simulink model "Old Observer"  (R2022a)
settings: Solver=VariableStepAuto  StartTime=0  StopTime=1000  RelTol=1e-3
undefined symbols (not defined in the file): A_HD, A_platform, B_HD, B_platform, C_HD, C_platform, E_platform, L_platform, P_platform, Q_platform
settings Model: Creator=ianam  LastModifiedBy=ianam
settings DebuggingCC: UnderSpecifiedDataTypeMsg=error  UnderSpecifiedDimensionMsg=error

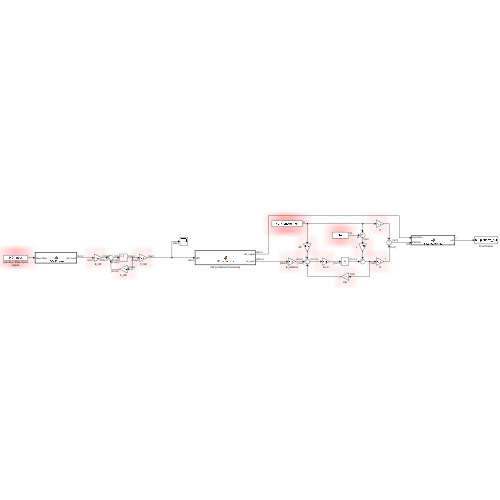
[thumbnail: Simulink's stored preview of the top-level diagram]
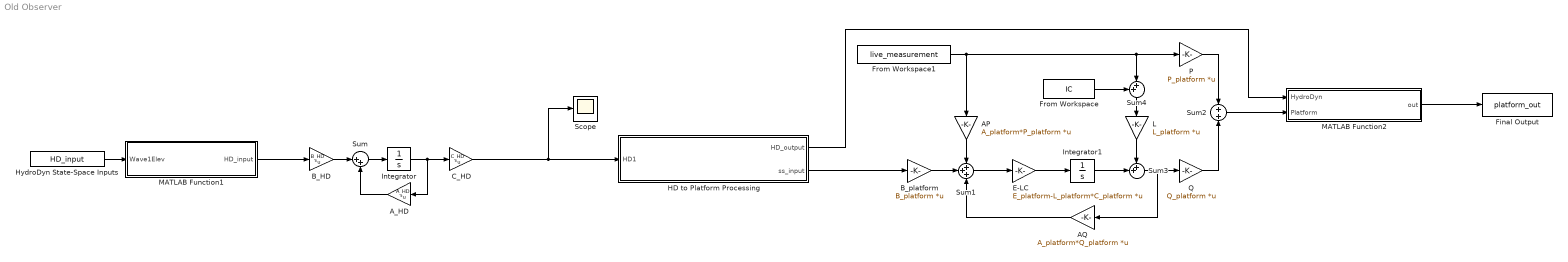
== system Old Observer ==
  AP : Gain  Gain=A_platform*P_platform  Multiplication=Matrix(K*u)
  AQ : Gain  Gain=A_platform*Q_platform  Multiplication=Matrix(K*u)
  A_HD : Gain  Gain=A_HD  Multiplication=Matrix(K*u)
  B_HD : Gain  Gain=B_HD  Multiplication=Matrix(K*u)
  B_platform : Gain  Gain=B_platform  Multiplication=Matrix(K*u)
  C_HD : Gain  Gain=C_HD  Multiplication=Matrix(K*u)
  E-LC : Gain  Gain=E_platform-L_platform*C_platform  Multiplication=Matrix(K*u)
  Final Output : ToWorkspace  VariableName=platform_out  SaveFormat=Timeseries  SampleTime=-1
  From Workspace : FromWorkspace  VariableName=IC
  From Workspace1 : FromWorkspace  VariableName=live_measurement
  HD to Platform Processing : MATLAB Function  TreatAsAtomicUnit=on
  HydroDyn State-Space Inputs : FromWorkspace  VariableName=HD_input
  Integrator : Integrator
  Integrator1 : Integrator
  L : Gain  Gain=L_platform  Multiplication=Matrix(K*u)
  MATLAB Function1 : MATLAB Function  TreatAsAtomicUnit=on
  MATLAB Function2 : MATLAB Function  TreatAsAtomicUnit=on
  P : Gain  Gain=P_platform  Multiplication=Matrix(K*u)
  Q : Gain  Gain=Q_platform  Multiplication=Matrix(K*u)
  Scope : Scope
  Sum : Sum  Inputs=|++
  Sum1 : Sum  Inputs=+++
  Sum2 : Sum  Inputs=+|+
  Sum3 : Sum  Inputs=++|
  Sum4 : Sum  Inputs=++|
  wires:
  Sum/1 -> Integrator/1
  Integrator/1 -> C_HD/1, A_HD/1
  A_HD/1 -> Sum/2
  B_HD/1 -> Sum/1
  MATLAB Function1/1(HD_input) -> B_HD/1
  HD to Platform Processing/2(ss_input) -> B_platform/1
  HydroDyn State-Space Inputs/1 -> MATLAB Function1/1(Wave1Elev)
  C_HD/1 -> Scope/1, HD to Platform Processing/1(HD1)
  AQ/1 -> Sum1/3
  B_platform/1 -> Sum1/2
  Sum1/1 -> E-LC/1
  E-LC/1 -> Integrator1/1
  AP/1 -> Sum1/1
  From Workspace1/1 -> P/1, Sum4/2, AP/1
  From Workspace/1 -> Sum4/1
  Integrator1/1 -> Sum3/2
  Sum4/1 -> L/1
  L/1 -> Sum3/1
  Sum3/1 -> AQ/1, Q/1
  P/1 -> Sum2/1
  Q/1 -> Sum2/2
  HD to Platform Processing/1(HD_output) -> MATLAB Function2/1(HydroDyn)
  Sum2/1 -> MATLAB Function2/2(Platform)
  MATLAB Function2/1(out) -> Final Output/1

== matlab function Old Observer/MATLAB Function1 ==
  data: Wave1Elev input; HD_input output
function HD_input = HDOutProcess(Wave1Elev)

% Create input vector
HD_input = zeros(37,1);

% Assign HD outputs to input vector
HD_input(37) = Wave1Elev;

end

== matlab function Old Observer/HD to Platform Processing ==
  data: HD_output output; HD1 input; ss_input output size=235,1
function [HD_output,ss_input] = HDOutProcess(HD1)

% Initialize
HydroF = zeros(6,1);
HD_output = zeros(25,1);

% Define quantities
Wave1Elev = HD1(1);
HydroF(1) = HD1(2);
HydroF(2) = HD1(3);
HydroF(3) = HD1(4);
HydroF(4) = HD1(5);
HydroF(5) = HD1(6);
HydroF(6) = HD1(7);

HD_output(:,1) = HD1(:);
HD_output(2:7) = HD_output(2:7);
HD_output(8:13) = HD_output(8:13);

% Create input vector
ss_input = zeros(235,1);

% Assign HD outputs to input vector
ss_input(40:45,1) = HydroF(:,1);

% ss_input(226,1) = Wave1Elev(1);

end

== matlab function Old Observer/MATLAB Function2 ==
  data: HydroDyn input; out output; Platform input
function out = passWaveForce(HydroDyn,Platform)

% Read Forces from HydroDyn Output
force = HydroDyn(2:end,1);

% Add Forces to Total Output
Platform(34:57,1) = force;

out = Platform;

end
